simulink model "Project1_4"  (R2017a)
settings: Solver=ode45  StartTime=0.0  StopTime=1  MaxStep=1e-4  RelTol=1e-3
values from neighbouring files (symbols this model uses):
  al = as*100    [Project1Var.m]
  ba = as*J/psi    [Project1Var.m]
  In = 20    [Project1Var.m]
  J = 0.001    [Project1Var.m]
  ki = ac^2*L    [Project1Var.m]
  kis = as^2*J/psi    [Project1Var.m]
  kp = ac*L    [Project1Var.m]
  kps = as*J/psi    [Project1Var.m]
  L = 2.5*10^(-3)    (= 0.0025)    [Project1Var.m]
  psi = 0.35    [Project1Var.m]
  R = 0.5    [Project1Var.m]
  Ra = ac*L-R    [Project1Var.m]
  Vn = 120    [Project1Var.m]
libraries: simulink x1
settings Model: Creator=Callum  LastModifiedBy=Callum

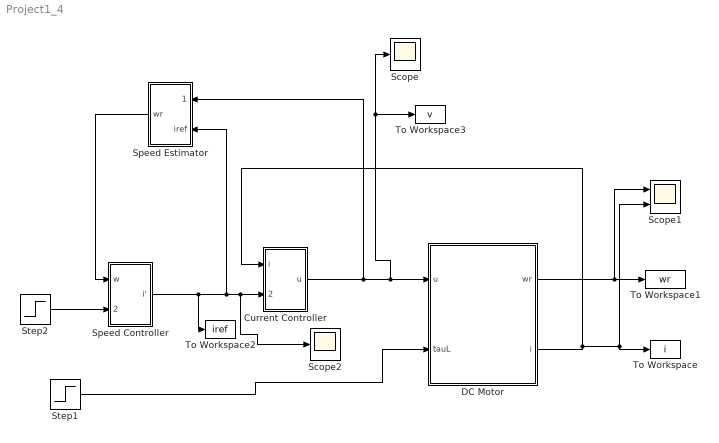
== system Project1_4 ==
  Current Controller : Subsystem
  DC Motor : Subsystem  mask{R=R, L=L, psi=psi, J=J}
      mask prompts: R "R (ohm)"; L "L (H)"; psi "psi(Vs)"; J "J (kgm^2)"
  Scope : Scope
  Scope1 : Scope  NumInputPorts=2
  Scope2 : Scope
  Speed Controller : Subsystem
  Speed Estimator : Subsystem
  Step1 : Step  Time=0.5  After=7  SampleTime=0
  Step2 : Step  Time=0.1  After=450  SampleTime=0
  To Workspace : ToWorkspace  VariableName=i  SaveFormat=Timeseries  SampleTime=-1
      settings: Save2DSignal=2-D array (concatenate along first dimension)
  To Workspace1 : ToWorkspace  VariableName=wr  SaveFormat=Timeseries  SampleTime=-1
      settings: Save2DSignal=2-D array (concatenate along first dimension)
  To Workspace2 : ToWorkspace  VariableName=iref  SaveFormat=Timeseries  SampleTime=-1
      settings: Save2DSignal=2-D array (concatenate along first dimension)
  To Workspace3 : ToWorkspace  VariableName=v  SaveFormat=Timeseries  SampleTime=-1
      settings: Save2DSignal=2-D array (concatenate along first dimension)
  wires:
  DC Motor/2(i) -> To Workspace/1, Scope1/2, Current Controller/1(i)
  DC Motor/1(wr) -> Scope1/1, To Workspace1/1
  Step1/1 -> DC Motor/2(tauL)
  Speed Controller/1(i') -> To Workspace2/1, Speed Estimator/2(iref), Scope2/1, Current Controller/2(i_ref)
  Step2/1 -> Speed Controller/2(w_ref)
  Speed Estimator/1(wr) -> Speed Controller/1(w)
  Current Controller/1(u) -> Speed Estimator/1(uref), To Workspace3/1, Scope/1, DC Motor/1(u)

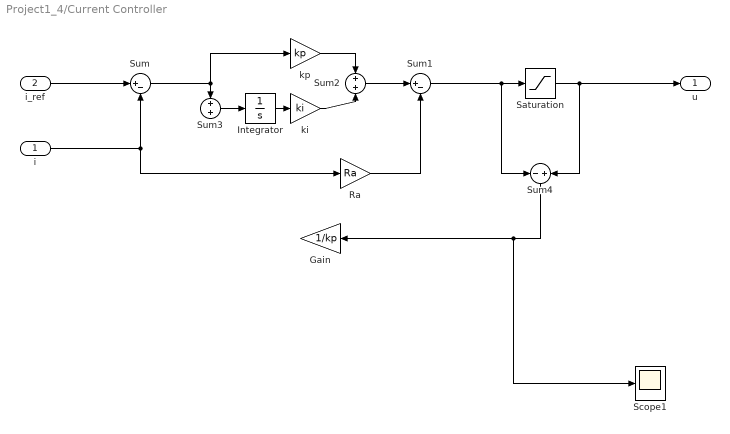
== system Project1_4/Current Controller ==
  i : Inport
  i_ref : Inport  Port=2
  Gain : Gain  Gain=1/kp
  Integrator : Integrator
  Ra : Gain  Gain=Ra
  Saturation : Saturate  UpperLimit=Vn  LowerLimit=-Vn
  Scope1 : Scope
  Sum : Sum  Inputs=|+-
  Sum1 : Sum  Inputs=|+-
  Sum2 : Sum
  Sum3 : Sum
  Sum4 : Sum  Inputs=-+
  ki : Gain  Gain=ki
  kp : Gain  Gain=kp
  u : Outport
  wires:
  Sum2/1 -> Sum1/1
  Sum1/1 -> Sum4/1, Saturation/1
  Ra/1 -> Sum1/2
  kp/1 -> Sum2/1
  ki/1 -> Sum2/2
  i/1 -> Ra/1, Sum/2
  i_ref/1 -> Sum/1
  Integrator/1 -> ki/1
  Sum/1 -> Sum3/1, kp/1
  Saturation/1 -> Sum4/2, u/1
  Sum3/1 -> Integrator/1
  Sum4/1 -> Scope1/1, Gain/1

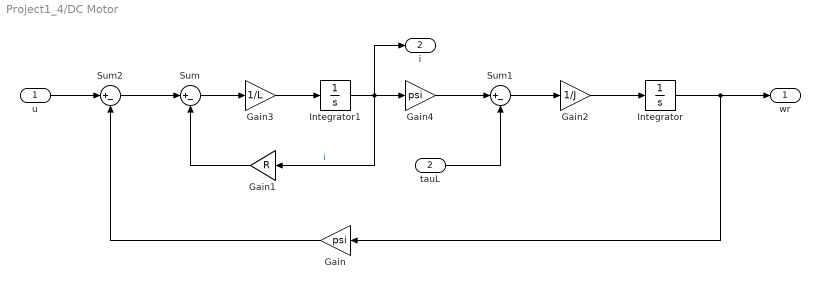
== system Project1_4/DC Motor ==
  u : Inport
  tauL : Inport  Port=2
  Gain : Gain  Gain=psi
  Gain1 : Gain  Gain=R
  Gain2 : Gain  Gain=1/J
  Gain3 : Gain  Gain=1/L
  Gain4 : Gain  Gain=psi
  Integrator : Integrator
  Integrator1 : Integrator
  Sum : Sum  Inputs=|+-
  Sum1 : Sum  Inputs=|+-
  Sum2 : Sum  Inputs=|+-
  wr : Outport
  i : Outport  Port=2
  wires:
  u/1 -> Sum2/1
  Integrator1/1 -> i/1, Gain1/1, Gain4/1  "i"
  Gain/1 -> Sum2/2
  tauL/1 -> Sum1/2
  Gain4/1 -> Sum1/1
  Integrator/1 -> wr/1, Gain/1
  Sum1/1 -> Gain2/1
  Gain2/1 -> Integrator/1
  Sum/1 -> Gain3/1
  Sum2/1 -> Sum/1
  Gain3/1 -> Integrator1/1
  Gain1/1 -> Sum/2

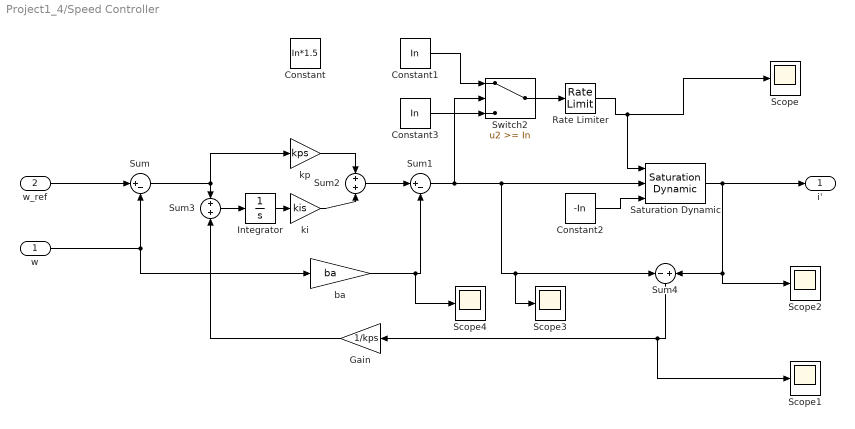
== system Project1_4/Speed Controller ==
  w : Inport
  w_ref : Inport  Port=2
  Constant : Constant  Value=In*1.5
  Constant1 : Constant  Value=In
  Constant2 : Constant  Value=-In
  Constant3 : Constant  Value=In
  Gain : Gain  Gain=1/kps
  Integrator : Integrator
  Rate Limiter : RateLimiter  RisingSlewLimit=100  FallingSlewLimit=-100  SampleTimeMode=inherited
  Saturation Dynamic : simulink/Discontinuities/Saturation Dynamic  OutMin=[]  OutMax=[]  OutDataTypeStr=Inherit: Same as second input  OutDataType=fixdt(1, 16)  OutScaling=2^-10  DoSatur=off
  Scope{,1..4} (5 alike) : Scope
  Sum : Sum  Inputs=|+-
  Sum1 : Sum  Inputs=|+-
  Sum2 : Sum
  Sum3 : Sum
  Sum4 : Sum  Inputs=-+
  Switch2 : Switch  Threshold=In
  ba : Gain  Gain=ba
  ki : Gain  Gain=kis
  kp : Gain  Gain=kps
  i' : Outport
  wires:
  Sum2/1 -> Sum1/1
  Sum1/1 -> Saturation Dynamic/2, Scope3/1, Sum4/1, Switch2/2
  kp/1 -> Sum2/1
  ki/1 -> Sum2/2
  w/1 -> ba/1, Sum/2
  w_ref/1 -> Sum/1
  Integrator/1 -> ki/1
  Sum/1 -> Sum3/1, kp/1
  Saturation Dynamic/1 -> Scope2/1, Sum4/2, i'/1
  Sum3/1 -> Integrator/1
  Sum4/1 -> Scope1/1, Gain/1
  Constant2/1 -> Saturation Dynamic/3
  Switch2/1 -> Rate Limiter/1
  Rate Limiter/1 -> Saturation Dynamic/1, Scope/1
  Constant3/1 -> Switch2/3
  Constant1/1 -> Switch2/1
  ba/1 -> Scope4/1, Sum1/2
  Gain/1 -> Sum3/2

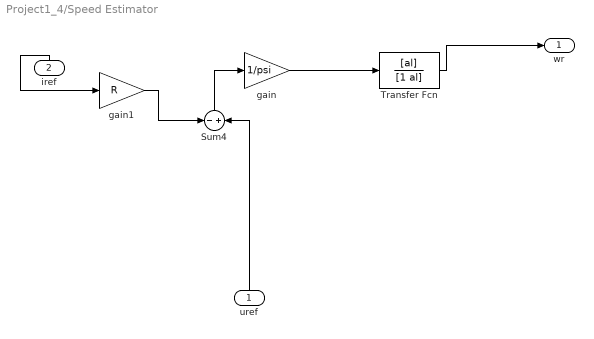
== system Project1_4/Speed Estimator ==
  uref : Inport
  iref : Inport  Port=2
  Sum4 : Sum  Inputs=-+
  Transfer Fcn : TransferFcn  Numerator=[al]  Denominator=[1 al]
  gain : Gain  Gain=1/psi
  gain1 : Gain  Gain=R
  wr : Outport
  wires:
  gain/1 -> Transfer Fcn/1
  gain1/1 -> Sum4/1
  Sum4/1 -> gain/1
  Transfer Fcn/1 -> wr/1
  uref/1 -> Sum4/2
  iref/1 -> gain1/1
